simulink library "BWB_library"  (R2017b)
settings: Solver=VariableStepAuto  StartTime=0.0  StopTime=10.0  RelTol=1e-3
undefined symbols (not defined in the file or in its folder): BWB, BWB_uncoupled, BWBlat, BWBlat1, BWBlon, F, I, Ixx, Iyy, Izz, Light, m, MIL, pqr0, ptp0, Vb0, x0, Xe0
libraries: aerolibasang x4, aerolibwind2 x3, shared6dof x2, aerolibadyn x2, aerolibatmos2 x1
(part 1 of 2)
settings Model: Creator=Liam Uni  LastModifiedBy=Liam Uni

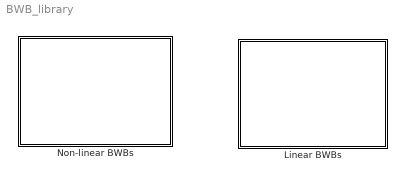
== system BWB_library ==
  Linear BWBs : Subsystem
      mask Display:
      | image('bwb.jpg');
      | 
      | disp('Linear')
  Non-linear BWBs : Subsystem
      mask Display:
      | image('bwb.jpg');
      | 
      | disp('Non-linear')

== system BWB_library/Linear BWBs ==
  BWB lateral : Subsystem  mask{x0=x0}
      mask prompts: x0 "Intial Conditions"
      mask init:
      | open('BWBss')
      mask DialogControl DescGroupVar Prompt: BWB lateral no engine
      mask DialogControl DescTextVar Prompt: Linear model of BWB's lateral dynamics, y(t)=[V p r phi psi] . 12 flaps.
      mask Display:
      | image('bwb.jpg');
      | port_label('input', 1, 'u(t)');
      | port_label('output', 1, 'y(t)');
  BWB lateral no engine : Subsystem  mask{x0=x0}
      mask prompts: x0 "Intial Conditions"
      mask init:
      | open('BWBss')
      mask DialogControl DescGroupVar Prompt: BWB lateral no engine
      mask DialogControl DescTextVar Prompt: Linear model of BWB's lateral dynamics, y(t)=[V p r phi psi] . 12 flaps.
      mask Display:
      | image('bwb.jpg');
      | port_label('input', 1, 'u(t)');
      | port_label('output', 1, 'y(t)');
  BWB linear : Subsystem  mask{x0=x0}
      mask prompts: x0 "Intial Conditions"
      mask init:
      | open('BWBss')
      mask DialogControl DescGroupVar Prompt: BWB linear
      mask DialogControl DescTextVar Prompt: Full State linear BWB, y(t)=[V p r phi psi U w q theta H]. 15 control inputs, 3 engines and 12 flaps
      mask Display:
      | image('bwb.jpg');
      | port_label('input', 1, 'u(t)');
      | port_label('output', 1, 'y(t)');
  BWB longitudinal : Subsystem  mask{x0=x0}
      mask prompts: x0 "Intial Conditions"
      mask init:
      | open('BWBss')
      mask DialogControl DescGroupVar Prompt: BWB longitudinal
      mask DialogControl DescTextVar Prompt: Linear model of BWB's longitudinal dynamics, y(t)=[U w q theta H] . 15 control inputs, 3 engines and 12 flaps.
      mask Display:
      | image('bwb.jpg');
      | port_label('input', 1, 'u(t)');
      | port_label('output', 1, 'y(t)');
  BWB longitudinal 1 engine : Subsystem  mask{x0=x0}
      mask prompts: x0 "Intial Conditions"
      mask init:
      | open('BWBss')
      mask DialogControl DescGroupVar Prompt: BWB longitudinal 1 engine
      mask DialogControl DescTextVar Prompt: Linear model of BWB's longitudinal dynamics, y(t)=[U w q theta H] . 13 control inputs, 1 engine and 12 flaps.
      mask Display:
      | image('bwb.jpg');
      | port_label('input', 1, 'u(t)');
      | port_label('output', 1, 'y(t)');
  BWB uncoupled : Subsystem  mask{x0=x0}
      mask prompts: x0 "Intial Conditions"
      mask init:
      | open('BWBss')
      mask DialogControl DescGroupVar Prompt: BWB linear uncoupled
      mask DialogControl DescTextVar Prompt: Full State linear BWB, y(t)=[V p r phi psi U w q theta H]. 15 control inputs, 3 engines and 12 flaps. Coupling terms between lateral and longitudinal dynamics are negated
      mask Display:
      | image('bwb.jpg');
      | port_label('input', 1, 'u(t)');
      | port_label('output', 1, 'y(t)');

== system BWB_library/Non-linear BWBs ==
  BWB non-linear : Subsystem  mask{Xe0=Xe0, Vb0=Vb0, ptp0=ptp0, pqr0=pqr0, m=m, I=I}
      mask prompts: Xe0 "Initial position in inertial axes [Xe, Ye, Ze]:"; Vb0 "Initial velocity in body axes [U,v,w]:"; ptp0 "Initial Euler orinetation [phi, theta, psi]:"; pqr0 "Initial body rotation rates [p,q,r]:"; m "Initial mass:"; I "Inertial matrix:"
      mask init:
      | % Mean Earth Radius
      | re=6371E3;
      | 
      | % Gravity 
      | g0=9.80665;
      | 
      | a=343;
      | 
      | Rho= 0.85;
      | 
      | %Gross Area/ m^2
      | Sgross= 1390.6;
      | 
      | %Sref/ m^2
      | Sref=   841.7;
      | 
      | %Wing span/ m
      | b=      80;
      | 
      | %Mean aerodynamic chord/ m
      | cbar=   12.31;
      | 
      | %Trapezoidal aspect ratio
      | AR=     7.14;
      | 
      | %Root chord/ m
      | Croot=  48;
      | 
      | %Tip chord/ m
      | Ctip=   4;
      | 
      | %CoG/ m
      | CoG=    29.4;
      | 
      | %Distance of engines from centre/m
      | Deng=5;
      | 
      | %Length of Aircraft/m
      | Length=50.9;
      | 
      | %% Normal Force Coefficient 
      | 
      | Cz0=    0.0217;
      | Czalf=  -5.4868;
      | Czf1=   -0.4866;
      | Czf2=   -0.1602;
      | Czf3=   -0.2222;
      | Czf4=   -0.2274;
      | Czf5=   -0.1042;
      | Czq=    -1.0787;
      | 
      | %% Axial Force Coefficient
      | 
      | Cx0=    0.0117;
      | Cx1=    -0.0200;
      | Cx2=    0.1200;
      | 
      | %% Side Force Coefficient
      | 
      | Cybet0=     -0.3086;
      | Cybetalf=   0.4879;
      | Cyp0=       -0.0814;
      | Cypalf=     2.0666;
      | Cyf1=       -0.0092;
      | Cyf2=       -0.0060;
      | Cyf3=       -0.0088;
      | Cyf4=       -0.0154;
      | Cyf5=       -0.0184;
      | Cydr=       0.0467;
      | Cyr=        -0.1555;
      | 
      | %% Roll Moment Coefficient
      | 
      | Clbet0=     -0.0465;
      | Clbetalf=   -0.3007;
      | Clp0=       -0.3562;
      | Clpalf=     0.0735;
      | Clf1=       -0.0274;
      | Clf2=       -0.0230;
      | Clf3=       -0.0442;
      | Clf4=       -0.0644;
      | Clf5=       -0.0396;
      | Cldr=       0.0156;
      | Clr0=       0.0272;
      | Clralf=     0.5867;
      | 
      | %% Pitch Moment Coefficient
      | 
      | Cm0=        -0.0370;
      | Cmalf=      -0.9950;
      | Cmq=        -0.8799;
      | Cmf1=       -0.3562;
      | Cmf2=       -0.1046;
      | Cmf3=       -0.1432;
      | Cmf4=       -0.1944;
      | Cmf5=       -0.1238;
      | 
      | %% Yaw Moment Coefficient
      | 
      | Cnbet0=    0.0152;
      | Cnbetalf=  -0.2787;
      | Cnp0=       0.0134;
      | Cnpalf=     -0.8733;
      | Cnr0=       -0.0315;
      | Cnralf=     0.0867;
      | Cnf1=       0.0016;
      | Cnf2=       0.0012;
      | Cnf3=       0.0014;
      | Cnf4=       0.0028;
      | Cnf5=       0.0042;
      | Cndr=       -0.0155;
      mask DialogControl DescGroupVar Prompt: BWB non-linear
      mask DialogControl DescTextVar Prompt: Non-linear full state linear BWB, y(t)=[V p r phi psi U w q theta H]. 15 control inputs, 3 engines and 12 flaps. With simplified environment
      mask Display:
      | image('bwb.jpg');
      | port_label('input', 1, 'u(t)');
      | port_label('output', 1, 'y(t)');
  BWB w/ environment : Subsystem  mask{Xe0=Xe0, Vb0=Vb0, ptp0=ptp0, pqr0=pqr0, m=m, I=I}
      mask prompts: Xe0 "Initial position in inertial axes [Xe, Ye, Ze]:"; Vb0 "Initial velocity in body axes [U,v,w]:"; ptp0 "Initial Euler orinetation [phi, theta, psi]:"; pqr0 "Initial body rotation rates [p,q,r]:"; m "Initial mass:"; I "Inertial matrix:"
      mask init:
      | %Gross Area/ m^2
      | Sgross= 1390.6;
      | 
      | %Sref/ m^2
      | Sref=   841.7;
      | 
      | %Wing span/ m
      | b=      80;
      | 
      | %Mean aerodynamic chord/ m
      | cbar=   12.31;
      | 
      | %Trapezoidal aspect ratio
      | AR=     7.14;
      | 
      | %Root chord/ m
      | Croot=  48;
      | 
      | %Tip chord/ m
      | Ctip=   4;
      | 
      | %CoG/ m
      | CoG=    29.4;
      | 
      | %Distance of engines from centre/m
      | Deng=5;
      | 
      | %Length of Aircraft/m
      | Length=50.9;
      | 
      | %% Normal Force Coefficient 
      | 
      | Cz0=    0.0217;
      | Czalf=  -5.4868;
      | Czf1=   -0.4866;
      | Czf2=   -0.1602;
      | Czf3=   -0.2222;
      | Czf4=   -0.2274;
      | Czf5=   -0.1042;
      | Czq=    -1.0787;
      | 
      | %% Axial Force Coefficient
      | 
      | Cx0=    0.0117;
      | Cx1=    -0.0200;
      | Cx2=    0.1200;
      | 
      | %% Side Force Coefficient
      | 
      | Cybet0=     -0.3086;
      | Cybetalf=   0.4879;
      | Cyp0=       -0.0814;
      | Cypalf=     2.0666;
      | Cyf1=       -0.0092;
      | Cyf2=       -0.0060;
      | Cyf3=       -0.0088;
      | Cyf4=       -0.0154;
      | Cyf5=       -0.0184;
      | Cydr=       0.0467;
      | Cyr=        -0.1555;
      | 
      | %% Roll Moment Coefficient
      | 
      | Clbet0=     -0.0465;
      | Clbetalf=   -0.3007;
      | Clp0=       -0.3562;
      | Clpalf=     0.0735;
      | Clf1=       -0.0274;
      | Clf2=       -0.0230;
      | Clf3=       -0.0442;
      | Clf4=       -0.0644;
      | Clf5=       -0.0396;
      | Cldr=       0.0156;
      | Clr0=       0.0272;
      | Clralf=     0.5867;
      | 
      | %% Pitch Moment Coefficient
      | 
      | Cm0=        -0.0370;
      | Cmalf=      -0.9950;
      | Cmq=        -0.8799;
      | Cmf1=       -0.3562;
      | Cmf2=       -0.1046;
      | Cmf3=       -0.1432;
      | Cmf4=       -0.1944;
      | Cmf5=       -0.1238;
      | 
      | %% Yaw Moment Coefficient
      | 
      | Cnbet0=    0.0152;
      | Cnbetalf=  -0.2787;
      | Cnp0=       0.0134;
      | Cnpalf=     -0.8733;
      | Cnr0=       -0.0315;
      | Cnralf=     0.0867;
      | Cnf1=       0.0016;
      | Cnf2=       0.0012;
      | Cnf3=       0.0014;
      | Cnf4=       0.0028;
      | Cnf5=       0.0042;
      | Cndr=       -0.0155;
      mask DialogControl DescGroupVar Prompt: BWB w/ environment
      mask DialogControl DescTextVar Prompt: Non-linear full state linear BWB, y(t)=[V p r phi psi U w q theta H]. 15 control inputs, 3 engines and 12 flaps. With realistic environment
      mask Display:
      | image('bwb.jpg');
      | port_label('input', 1, 'u(t)');
      | port_label('output', 1, 'y(t)');

== system BWB_library/Linear BWBs/BWB lateral ==
  u(t) : Inport
  State-Space : StateSpace  A=BWBlat.A  B=BWBlat.B  C=BWBlat.C  D=BWBlat.D  InitialCondition=x0
  System States : Outport
  wires:
  State-Space/1 -> System States/1
  u(t)/1 -> State-Space/1

== system BWB_library/Linear BWBs/BWB lateral no engine ==
  u(t) : Inport
  State-Space : StateSpace  A=BWBlat1.A  B=BWBlat1.B  C=BWBlat1.C  D=BWBlat1.D  InitialCondition=x0
  System States : Outport
  wires:
  u(t)/1 -> State-Space/1
  State-Space/1 -> System States/1

== system BWB_library/Linear BWBs/BWB linear ==
  u(t) : Inport
  State-Space : StateSpace  A=BWB.A  B=BWB.B  C=BWB.C  D=BWB.D  InitialCondition=x0
  System States : Outport
  wires:
  State-Space/1 -> System States/1
  u(t)/1 -> State-Space/1

== system BWB_library/Linear BWBs/BWB longitudinal ==
  u(t) : Inport
  State-Space : StateSpace  A=BWBlon.A  B=BWBlon.B  C=BWBlon.C  D=BWBlon.D  InitialCondition=x0
  System States : Outport
  wires:
  u(t)/1 -> State-Space/1
  State-Space/1 -> System States/1

== system BWB_library/Linear BWBs/BWB longitudinal 1 engine ==
  u(t) : Inport
  State-Space : StateSpace  A=BWBlon.A  B=BWBlon.B  C=BWBlon.C  D=BWBlon.D  InitialCondition=x0
  System States : Outport
  wires:
  u(t)/1 -> State-Space/1
  State-Space/1 -> System States/1

== system BWB_library/Linear BWBs/BWB uncoupled ==
  u(t) : Inport
  State-Space : StateSpace  A=BWB_uncoupled.A  B=BWB_uncoupled.B  C=BWB_uncoupled.C  D=BWB_uncoupled.D  InitialCondition=x0
  System States : Outport
  wires:
  State-Space/1 -> System States/1
  u(t)/1 -> State-Space/1

== system BWB_library/Non-linear BWBs/BWB non-linear ==
  u(t) : Inport
  6DOF (Euler Angles) : shared6dof/6DOF (Euler Angles)  units=Metric (MKS)  mtype=Fixed  rep=Euler Angles  xme_0=Xe0  Vm_0=Vb0  eul_0=ptp0*0.0174533  pm_0=pqr0*0.0174533  mass_0=m  mass_e=0.5  mass_f=2.0  inertia=diag([Ixx, Iyy, Izz])  inertia_e=eye(3)  inertia_f=2*eye(3)  k_quat=1.0  vre_flag=on  abi_flag=on
      settings: SourceProductBaseCode=AE
  Bus Selector1 : BusSelector  OutputSignals=Vb,phi;theta;psi,pqr,Xe
  Demux : Demux  Outputs=3
  Demux1 : Demux  Outputs=3
  Demux2 : Demux  Outputs=3
  Gain : Gain  Gain=-1
  Model o/p bus : BusCreator  Inputs=6
  Mux : Mux  Inputs=10
  Selector : Selector  InputPortWidth=3  IndexOptions=Index vector (dialog)  Indices=[3]  OutputSizes=1
  Subsystem1 : Subsystem
  Subsystem3 : Subsystem
  Terminator1 : Terminator
  Terminator2 : Terminator
  Terminator3 : Terminator
  System States : Outport
  wires:
  6DOF (Euler Angles)/1 -> Model o/p bus/1  "Ve"
  6DOF (Euler Angles)/7 -> Terminator2/1
  6DOF (Euler Angles)/9 -> Terminator3/1
  6DOF (Euler Angles)/3 -> Model o/p bus/3  "phi;theta;psi"
  6DOF (Euler Angles)/6 -> Model o/p bus/6  "pqr"
  6DOF (Euler Angles)/4 -> Model o/p bus/4  "DCM"
  6DOF (Euler Angles)/8 -> Terminator1/1
  6DOF (Euler Angles)/5 -> Model o/p bus/5  "Vb"
  6DOF (Euler Angles)/2 -> Model o/p bus/2  "Xe"
  Subsystem3/1(Forces) -> 6DOF (Euler Angles)/1
  Subsystem3/2(Moments) -> 6DOF (Euler Angles)/2
  Subsystem1/1(Environment) -> Subsystem3/2(Environment)
  u(t)/1 -> Subsystem3/1(ud(t))
  Bus Selector1/2 -> Demux1/1  "<phi;theta;psi>"
  Mux/1 -> System States/1
  Demux/1 -> Mux/6
  Demux2/2 -> Mux/8
  Demux2/3 -> Mux/3
  Bus Selector1/3 -> Demux2/1  "<pqr>"
  Bus Selector1/1 -> Demux/1  "<Vb>"
  Model o/p bus/1 -> Bus Selector1/1, Subsystem1/1(System States)
  Demux/3 -> Mux/7
  Demux1/3 -> Mux/5
  Gain/1 -> Mux/10
  Demux1/1 -> Mux/4
  Demux2/1 -> Mux/2
  Demux/2 -> Mux/1
  Demux1/2 -> Mux/9
  Selector/1 -> Gain/1
  Bus Selector1/4 -> Selector/1  "<Xe>"

== system BWB_library/Non-linear BWBs/BWB w// environment ==
  u(t) : Inport
  6DOF (Euler Angles) : shared6dof/6DOF (Euler Angles)  units=Metric (MKS)  mtype=Fixed  rep=Euler Angles  xme_0=Xe0  Vm_0=Vb0  eul_0=ptp0*0.0174533  pm_0=pqr0*0.0174533  mass_0=m  mass_e=0.5  mass_f=2.0  inertia=diag([Ixx, Iyy, Izz])  inertia_e=eye(3)  inertia_f=2*eye(3)  k_quat=1.0  vre_flag=on  abi_flag=on
      settings: SourceProductBaseCode=AE
  Bus Selector1 : BusSelector  OutputSignals=Vb,phi;theta;psi,pqr,Xe
  Demux : Demux  Outputs=3
  Demux1 : Demux  Outputs=3
  Demux2 : Demux  Outputs=3
  Gain : Gain  Gain=-1
  Model o/p bus : BusCreator  Inputs=6
  Mux : Mux  Inputs=10
  Selector : Selector  InputPortWidth=3  IndexOptions=Index vector (dialog)  Indices=[3]  OutputSizes=1
  Subsystem1 : Subsystem
  Subsystem3 : Subsystem
  Terminator1 : Terminator
  Terminator2 : Terminator
  Terminator3 : Terminator
  System States : Outport
  wires:
  6DOF (Euler Angles)/1 -> Model o/p bus/1  "Ve"
  6DOF (Euler Angles)/7 -> Terminator2/1
  6DOF (Euler Angles)/9 -> Terminator3/1
  6DOF (Euler Angles)/3 -> Model o/p bus/3  "phi;theta;psi"
  6DOF (Euler Angles)/6 -> Model o/p bus/6  "pqr"
  6DOF (Euler Angles)/4 -> Model o/p bus/4  "DCM"
  6DOF (Euler Angles)/8 -> Terminator1/1
  6DOF (Euler Angles)/5 -> Model o/p bus/5  "Vb"
  6DOF (Euler Angles)/2 -> Model o/p bus/2  "Xe"
  Subsystem3/1(Forces) -> 6DOF (Euler Angles)/1
  Subsystem3/2(Moments) -> 6DOF (Euler Angles)/2
  Subsystem1/1(Environment) -> Subsystem3/2(Environment)
  u(t)/1 -> Subsystem3/1(ud(t))
  Bus Selector1/2 -> Demux1/1  "<phi;theta;psi>"
  Demux2/3 -> Mux/3
  Demux2/1 -> Mux/2
  Model o/p bus/1 -> Bus Selector1/1, Subsystem1/1(System States)
  Demux2/2 -> Mux/8
  Demux1/2 -> Mux/9
  Bus Selector1/1 -> Demux/1  "<Vb>"
  Bus Selector1/3 -> Demux2/1  "<pqr>"
  Demux1/1 -> Mux/4
  Demux/2 -> Mux/1
  Demux/3 -> Mux/7
  Demux/1 -> Mux/6
  Demux1/3 -> Mux/5
  Bus Selector1/4 -> Selector/1  "<Xe>"
  Selector/1 -> Gain/1
  Mux/1 -> System States/1
  Gain/1 -> Mux/10

== system BWB_library/Non-linear BWBs/BWB non-linear/Subsystem1 ==
  System States : Inport
  Abs : Abs
  Bus Creator : BusCreator  Inputs=7
  Bus Selector1 : BusSelector  OutputSignals=Xe,phi;theta;psi,DCM,Vb,pqr
  Constant : Constant  Value=0
  Constant2 : Constant  Value=Rho
  Gain : Gain  Gain=0.5
  Gravity in Earth Axes : Gain  Gain=m  SaturateOnIntegerOverflow=on  OutDataTypeStr=Inherit: Same as input  ParamDataTypeStr=Inherit: Same as input
  Height : Selector  InputPortWidth=3  IndexOptions=Index vector (dialog)  Indices=[3]  OutputSizes=1
  "Incidence, Sideslip, & Airspeed" : aerolibasang/Incidence, Sideslip, & Airspeed
      settings: SourceProductName=Aerospace Blockset
  Inertial to Body : Product  Multiplication=Matrix(*)  SaturateOnIntegerOverflow=on  InputSameDT=on  OutDataTypeStr=Inherit: Same as first input
  Math Function : Math  Operator=square  SaturateOnIntegerOverflow=on
  Mux : Mux  Inputs=3
  Mux1 : Mux  Inputs=2
  Product : Product
  Selector : Selector  InputPortWidth=3  IndexOptions=Index vector (dialog)  Indices=[3]  OutputSizes=1
  Subsystem1 : Subsystem
  z-->h : Abs  SaturateOnIntegerOverflow=on
  Environment : Outport
  wires:
  Bus Selector1/3 -> Inertial to Body/1  "<DCM>"
  Bus Selector1/2 -> Bus Creator/3  "<phi;theta;psi>"
  Bus Creator/1 -> Environment/1
  Selector/1 -> Abs/1
  Abs/1 -> Bus Creator/7  "Altitude"
  z-->h/1 -> Subsystem1/1(Height)
  Gain/1 -> Product/1
  Product/1 -> Bus Creator/6  "qbar"
  Constant/1 -> Mux/1, Mux/2
  Gravity in Earth Axes/1 -> Mux/3
  Math Function/1 -> Product/2
  Constant2/1 -> Gain/1  "rho"
  Bus Selector1/1 -> Height/1, Selector/1  "<Xe>"
  Height/1 -> z-->h/1
  Mux/1 -> Inertial to Body/2
  Subsystem1/1(g) -> Gravity in Earth Axes/1
  Inertial to Body/1 -> Bus Creator/2  "Fg"
  Bus Selector1/4 -> "Incidence, Sideslip, & Airspeed"/1  "<Vb>"
  Bus Selector1/5 -> Bus Creator/1  "<pqr>"
  "Incidence, Sideslip, & Airspeed"/1 -> Mux1/1
  "Incidence, Sideslip, & Airspeed"/2 -> Mux1/2
  Mux1/1 -> Bus Creator/5  "Incid"
  "Incidence, Sideslip, & Airspeed"/3 -> Bus Creator/4, Math Function/1  "V"
  System States/1 -> Bus Selector1/1

== system BWB_library/Non-linear BWBs/BWB non-linear/Subsystem3 ==
  ud(t) : Inport
  Environment : Inport  Port=2
  Bus Selector : BusSelector  OutputSignals=Incid,V,pqr,qbar,Fg
  Forces and Moments : Subsystem  AncestorBlock=aeroblk_lib_HL20/HL20 Airframe/Forces and Moments
  Subsystem : Subsystem
  Subsystem2 : Subsystem
  Sum : Sum  Inputs=|++  SaturateOnIntegerOverflow=on  InputSameDT=on  OutDataTypeStr=Inherit: Same as first input
  Forces : Outport
  Moments : Outport  Port=2
  wires:
  ud(t)/1 -> Subsystem2/1(Control Inputs)
  Bus Selector/5 -> Sum/2  "<Fg>"
  Subsystem/1(Aerodynamic Coeffs) -> Forces and Moments/1(Coeff)
  Forces and Moments/1(X,Y,Z) -> Sum/1
  Forces and Moments/2(LMN) -> Moments/1
  Sum/1 -> Forces/1
  Environment/1 -> Bus Selector/1
  Bus Selector/1 -> Subsystem/2(incid)  "<Incid>"
  Bus Selector/2 -> Subsystem/3(V)  "<V>"
  Bus Selector/3 -> Subsystem/4(pqr)  "<pqr>"
  Bus Selector/4 -> Forces and Moments/3(qbar)  "<qbar>"
  Subsystem2/1(Aerodynamic Controls) -> Subsystem/1(u(t))
  Subsystem2/2(Engine Controls) -> Forces and Moments/2(Thrust)

== system BWB_library/Non-linear BWBs/BWB w// environment/Subsystem1 ==
  System States : Inport
  Abs : Abs
  Alpha,Beta,Mach1 : Subsystem
  Bus Creator : BusCreator  Inputs=7
  Bus Selector1 : BusSelector  OutputSignals=Ve,Xe,phi;theta;psi,DCM,Vb,pqr
  Environment Models1 : Subsystem
  Selector : Selector  InputPortWidth=3  IndexOptions=Index vector (dialog)  Indices=[3]  OutputSizes=1
  Environment : Outport
  wires:
  Alpha,Beta,Mach1/3(V) -> Bus Creator/4  "V"
  Alpha,Beta,Mach1/2("p,q,r ") -> Bus Creator/3  "pqr"
  Bus Selector1/6 -> Alpha,Beta,Mach1/6(p,q,r)  "<pqr>"
  Bus Selector1/2 -> Selector/1, Environment Models1/2(Xe)  "<Xe>"
  Alpha,Beta,Mach1/4(Mach) -> Bus Creator/5  "Mach"
  Bus Selector1/1 -> Environment Models1/1(Ve)  "<Ve>"
  Bus Selector1/4 -> Environment Models1/4(DCM)  "<DCM>"
  Environment Models1/4(Air Density) -> Alpha,Beta,Mach1/3(Air Density)
  System States/1 -> Bus Selector1/1
  Environment Models1/2(Speed of Sound) -> Alpha,Beta,Mach1/1(Speed of Sound)
  Bus Selector1/3 -> Environment Models1/3(Euler)  "<phi;theta;psi>"
  Environment Models1/1(Fg) -> Bus Creator/1  "Fg"
  Alpha,Beta,Mach1/1(qbar) -> Bus Creator/2  "qbar"
  Bus Creator/1 -> Environment/1
  Alpha,Beta,Mach1/5(Incid) -> Bus Creator/6  "Incid"
  Environment Models1/5(Wind Angular Rates) -> Alpha,Beta,Mach1/4(Wind Angular Rates)
  Bus Selector1/5 -> Alpha,Beta,Mach1/5(Vb)  "<Vb>"
  Environment Models1/3(Wind Velocity) -> Alpha,Beta,Mach1/2(Wind Velocity)
  Selector/1 -> Abs/1
  Abs/1 -> Bus Creator/7  "Altitude"

== system BWB_library/Non-linear BWBs/BWB w// environment/Subsystem3 ==
  ud(t) : Inport
  Environment : Inport  Port=2
  Bus Selector : BusSelector  OutputSignals=Incid,V,pqr,qbar,Fg
  Forces and Moments : Subsystem  AncestorBlock=aeroblk_lib_HL20/HL20 Airframe/Forces and Moments
  Subsystem : Subsystem
  Subsystem2 : Subsystem
  Sum : Sum  Inputs=|++  SaturateOnIntegerOverflow=on  InputSameDT=on  OutDataTypeStr=Inherit: Same as first input
  Forces : Outport
  Moments : Outport  Port=2
  wires:
  ud(t)/1 -> Subsystem2/1(Control Inputs)
  Bus Selector/5 -> Sum/2  "<Fg>"
  Subsystem/1(Aerodynamic Coeffs) -> Forces and Moments/1(Coeff)
  Forces and Moments/1(X,Y,Z) -> Sum/1
  Forces and Moments/2(LMN) -> Moments/1
  Sum/1 -> Forces/1
  Environment/1 -> Bus Selector/1
  Bus Selector/1 -> Subsystem/2(incid)  "<Incid>"
  Bus Selector/2 -> Subsystem/3(V)  "<V>"
  Bus Selector/3 -> Subsystem/4(pqr)  "<pqr>"
  Bus Selector/4 -> Forces and Moments/3(qbar)  "<qbar>"
  Subsystem2/1(Aerodynamic Controls) -> Subsystem/1(u(t))
  Subsystem2/2(Engine Controls) -> Forces and Moments/2(Thrust)

== system BWB_library/Non-linear BWBs/BWB non-linear/Subsystem1/Subsystem1 ==
  Height : Inport
  Add : Sum
  Constant1 : Constant  Value=re
  Constant3 : Constant  Value=g0
  Divide : Product  Inputs=*/
  Product1 : Product
  Square : Math  Operator=square  RndMeth=Zero  SaturateOnIntegerOverflow=on
  g : Outport
  wires:
  Add/1 -> Divide/2
  Constant1/1 -> Divide/1, Add/1
  Square/1 -> Product1/1
  Divide/1 -> Square/1
  Product1/1 -> g/1
  Constant3/1 -> Product1/2
  Height/1 -> Add/2

== system BWB_library/Non-linear BWBs/BWB non-linear/Subsystem3/Forces and Moments ==
  Coeff : Inport
  Thrust : Inport  Port=2  Unit=N
  qbar : Inport  Port=3  Unit=Pa
  Aerodynamic Forces and Moments : aerolibadyn/Aerodynamic Forces and Moments   inputAxes=Body  outputForceAxes=Body  outputMomentAxes=Body  S=Sref  b=b  cbar=Croot
      settings: SourceProductName=Aerospace Blockset
  Constant1 : Constant  Value=[(CoG+8), 0, 0]'
  Constant3 : Constant  Value=[CoG 0, 0]'
  Subsystem3 : Subsystem
  Sum : Sum  Inputs=++|  SaturateOnIntegerOverflow=on  InputSameDT=on  OutDataTypeStr=Inherit: Same as first input
  Sum1 : Sum  Inputs=++|  SaturateOnIntegerOverflow=on  InputSameDT=on  OutDataTypeStr=Inherit: Same as first input
  X,Y,Z : Outport  Unit=N  InitialOutput=0
  LMN : Outport  Port=2  Unit=N*m  InitialOutput=0
  wires:
  Constant1/1 -> Aerodynamic Forces and Moments/4
  Constant3/1 -> Aerodynamic Forces and Moments/3
  Aerodynamic Forces and Moments/1 -> Sum/2
  Aerodynamic Forces and Moments/2 -> Sum1/2
  Sum/1 -> X,Y,Z/1
  qbar/1 -> Aerodynamic Forces and Moments/2
  Coeff/1 -> Aerodynamic Forces and Moments/1
  Thrust/1 -> Subsystem3/1(Thrust)
  Subsystem3/1(Engine Forces) -> Sum/1
  Sum1/1 -> LMN/1
  Subsystem3/2(Engine Moments) -> Sum1/1

== system BWB_library/Non-linear BWBs/BWB non-linear/Subsystem3/Subsystem ==
  u(t) : Inport
  incid : Inport  Port=2
  V : Inport  Port=3
  pqr : Inport  Port=4
  Demux : Demux  Outputs=2
  Mux : Mux  Inputs=2
  Subsystem3 : Subsystem
  Subsystem4 : Subsystem
  Aerodynamic Coeffs : Outport
  wires:
  u(t)/1 -> Subsystem4/1(u(t)), Subsystem3/1(u(t))
  Subsystem3/1(Force Coefficients) -> Mux/1
  Mux/1 -> Aerodynamic Coeffs/1
  Subsystem4/1(Moment Coefficients) -> Mux/2
  V/1 -> Subsystem4/2(V), Subsystem3/2(V)
  Demux/1 -> Subsystem4/3(Alpha), Subsystem3/3(Alpha)
  Demux/2 -> Subsystem4/4(Beta), Subsystem3/4(Beta)
  pqr/1 -> Subsystem3/5(pqr), Subsystem4/5(pqr)
  incid/1 -> Demux/1

== system BWB_library/Non-linear BWBs/BWB non-linear/Subsystem3/Subsystem2 ==
  Control Inputs : Inport
  Demux : Demux  Outputs=15
  Mux : Mux  Inputs=12
  Mux1 : Mux  Inputs=3
  Aerodynamic Controls : Outport
  Engine Controls : Outport  Port=2
  wires:
  Control Inputs/1 -> Demux/1
  Mux/1 -> Aerodynamic Controls/1
  Demux/9 -> Mux/9
  Demux/7 -> Mux/7
  Demux/8 -> Mux/8
  Demux/12 -> Mux/12
  Demux/1 -> Mux/1
  Demux/10 -> Mux/10
  Demux/11 -> Mux/11
  Demux/3 -> Mux/3
  Demux/6 -> Mux/6
  Demux/4 -> Mux/4
  Demux/2 -> Mux/2
  Demux/5 -> Mux/5
  Demux/13 -> Mux1/1
  Demux/14 -> Mux1/2
  Demux/15 -> Mux1/3
  Mux1/1 -> Engine Controls/1

== system BWB_library/Non-linear BWBs/BWB w// environment/Subsystem1/Alpha,Beta,Mach1 ==
  Speed of Sound : Inport  Unit=m/s
  Wind Velocity : Inport  Port=2  Unit=m/s  PortDimensions=3
  Air Density : Inport  Port=3  Unit=kg/m^3
  Wind Angular Rates : Inport  Port=4  Unit=rad/s  PortDimensions=3
  Vb : Inport  Port=5  Unit=m/second  PortDimensions=3
  p,q,r : Inport  Port=6  Unit=rad/s  PortDimensions=3
  Dynamic Pressure : aerolibasang/Dynamic Pressure
  "Incidence, Sideslip & Airspeed" : aerolibasang/Incidence, Sideslip, & Airspeed
      settings: SourceProductName=Aerospace Blockset
  Mach Number : aerolibasang/Mach Number
      settings: SourceProductName=Aerospace Blockset  SourceProductBaseCode=AE
  Mux : Mux  Inputs=2
  Sum : Sum  Inputs=|+-  SaturateOnIntegerOverflow=on  InputSameDT=on  OutDataTypeStr=Inherit: Same as first input
  Sum1 : Sum  Inputs=|++  SaturateOnIntegerOverflow=on  InputSameDT=on  OutDataTypeStr=Inherit: Same as first input
  qbar : Outport  Unit=Pa  InitialOutput=0
  "p,q,r " : Outport  Port=2  Unit=rad/s
  V : Outport  Port=3  Unit=m/s
  Mach : Outport  Port=4
  Incid : Outport  Port=5  Unit=rad
  wires:
  "Incidence, Sideslip & Airspeed"/3 -> V/1
  Dynamic Pressure/1 -> qbar/1
  Air Density/1 -> Dynamic Pressure/2
  Mach Number/1 -> Mach/1
  Sum/1 -> Dynamic Pressure/1, Mach Number/1, "Incidence, Sideslip & Airspeed"/1
  Vb/1 -> Sum/1
  Speed of Sound/1 -> Mach Number/2
  Wind Velocity/1 -> Sum/2
  "Incidence, Sideslip & Airspeed"/2 -> Mux/2  "Beta"
  Mux/1 -> Incid/1
  "Incidence, Sideslip & Airspeed"/1 -> Mux/1  "Alpha"
  p,q,r/1 -> Sum1/1
  Wind Angular Rates/1 -> Sum1/2
  Sum1/1 -> "p,q,r "/1

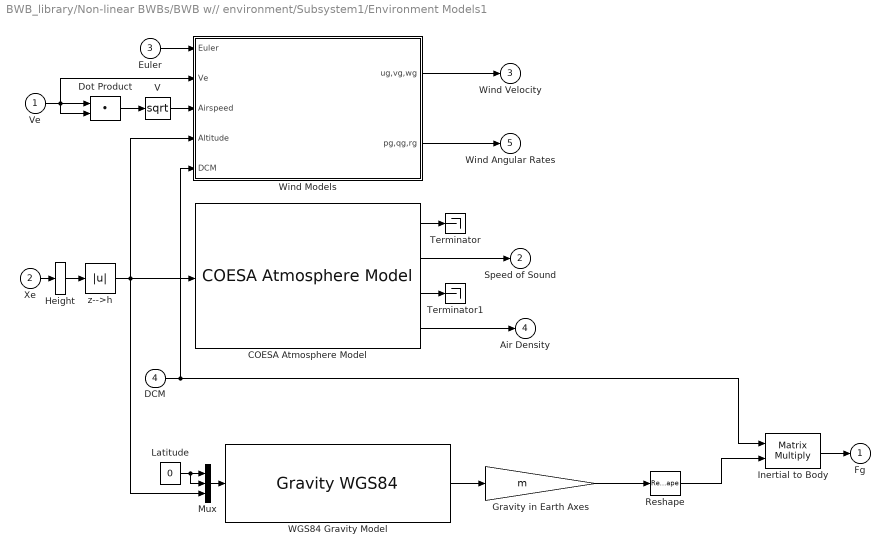
== system BWB_library/Non-linear BWBs/BWB w// environment/Subsystem1/Environment Models1 ==
  Ve : Inport  Unit=m/s
  Xe : Inport  Port=2  Unit=meter  PortDimensions=3
  Euler : Inport  Port=3  Unit=rad
  DCM : Inport  Port=4
  COESA Atmosphere Model : aerolibatmos2/COESA Atmosphere Model  units=Metric (MKS)  spec=1976 COESA-extended U.S. Standard Atmosphere  model=Profile  profile_var=High temperature  profile_percent=10%  profile_alt=5 km (16404 ft)  envelope_var=High temperature  envelope_percent=1%  action=None
  Dot Product : DotProduct  SaturateOnIntegerOverflow=on  OutDataTypeStr=Inherit: Inherit via internal rule
  Gravity in Earth Axes : Gain  Gain=m  SaturateOnIntegerOverflow=on  OutDataTypeStr=Inherit: Same as input  ParamDataTypeStr=Inherit: Same as input
  Height : Selector  InputPortWidth=3  IndexOptions=Index vector (dialog)  Indices=[3]  OutputSizes=1
  Inertial to Body : Product  Multiplication=Matrix(*)  SaturateOnIntegerOverflow=on  InputSameDT=on  OutDataTypeStr=Inherit: Same as first input
  Latitude : Constant  Value=0
  Mux : Mux  Inputs=3
  Reshape : Reshape
  Terminator : Terminator
  Terminator1 : Terminator
  V : Math  Operator=sqrt  SaturateOnIntegerOverflow=on
  "WGS84 Gravity Model  " : GravityWGS84  action=None
  Wind Models : Subsystem
  z-->h : Abs  SaturateOnIntegerOverflow=on
  Fg : Outport  Unit=N  InitialOutput=0
  Speed of Sound : Outport  Port=2  Unit=m/second  InitialOutput=0
  Wind Velocity : Outport  Port=3  Unit=m/second  InitialOutput=0
  Air Density : Outport  Port=4  Unit=kg/m^3  InitialOutput=0
  Wind Angular Rates : Outport  Port=5  Unit=rad/second  InitialOutput=0
  wires:
  Mux/1 -> "WGS84 Gravity Model  "/1
  Euler/1 -> Wind Models/1(Euler)
  Ve/1 -> Dot Product/2, Wind Models/2(Ve), Dot Product/1
  Wind Models/1(ug,vg,wg) -> Wind Velocity/1
  Wind Models/2(pg,qg,rg) -> Wind Angular Rates/1
  Dot Product/1 -> V/1
  z-->h/1 -> Mux/3, COESA Atmosphere Model/1, Wind Models/4(Altitude)
  COESA Atmosphere Model/4 -> Air Density/1
  COESA Atmosphere Model/2 -> Speed of Sound/1
  COESA Atmosphere Model/3 -> Terminator1/1
  COESA Atmosphere Model/1 -> Terminator/1
  Height/1 -> z-->h/1
  Xe/1 -> Height/1
  Latitude/1 -> Mux/2, Mux/1
  "WGS84 Gravity Model  "/1 -> Gravity in Earth Axes/1
  DCM/1 -> Wind Models/5(DCM), Inertial to Body/1
  Inertial to Body/1 -> Fg/1
  V/1 -> Wind Models/3(Airspeed)
  Reshape/1 -> Inertial to Body/2
  Gravity in Earth Axes/1 -> Reshape/1

== system BWB_library/Non-linear BWBs/BWB w// environment/Subsystem3/Forces and Moments ==
  Coeff : Inport
  Thrust : Inport  Port=2  Unit=N
  qbar : Inport  Port=3  Unit=Pa
  Aerodynamic Forces and Moments : aerolibadyn/Aerodynamic Forces and Moments   inputAxes=Body  outputForceAxes=Body  outputMomentAxes=Body  S=Sref  b=b  cbar=Croot
      settings: SourceProductName=Aerospace Blockset
  Constant1 : Constant  Value=[(CoG+8), 0, 0]'
  Constant3 : Constant  Value=[CoG 0, 0]'
  Subsystem3 : Subsystem
  Sum : Sum  Inputs=++|  SaturateOnIntegerOverflow=on  InputSameDT=on  OutDataTypeStr=Inherit: Same as first input
  Sum1 : Sum  Inputs=++|  SaturateOnIntegerOverflow=on  InputSameDT=on  OutDataTypeStr=Inherit: Same as first input
  X,Y,Z : Outport  Unit=N  InitialOutput=0
  LMN : Outport  Port=2  Unit=N*m  InitialOutput=0
  wires:
  Constant1/1 -> Aerodynamic Forces and Moments/4
  Constant3/1 -> Aerodynamic Forces and Moments/3
  Aerodynamic Forces and Moments/1 -> Sum/2
  Aerodynamic Forces and Moments/2 -> Sum1/2
  Sum/1 -> X,Y,Z/1
  qbar/1 -> Aerodynamic Forces and Moments/2
  Coeff/1 -> Aerodynamic Forces and Moments/1
  Thrust/1 -> Subsystem3/1(Thrust)
  Subsystem3/1(Engine Forces) -> Sum/1
  Sum1/1 -> LMN/1
  Subsystem3/2(Engine Moments) -> Sum1/1

== system BWB_library/Non-linear BWBs/BWB w// environment/Subsystem3/Subsystem ==
  u(t) : Inport
  incid : Inport  Port=2
  V : Inport  Port=3
  pqr : Inport  Port=4
  Demux : Demux  Outputs=2
  Mux : Mux  Inputs=2
  Subsystem3 : Subsystem
  Subsystem4 : Subsystem
  Aerodynamic Coeffs : Outport
  wires:
  u(t)/1 -> Subsystem4/1(u(t)), Subsystem3/1(u(t))
  Subsystem3/1(Force Coefficients) -> Mux/1
  Mux/1 -> Aerodynamic Coeffs/1
  Subsystem4/1(Moment Coefficients) -> Mux/2
  V/1 -> Subsystem4/2(V), Subsystem3/2(V)
  Demux/1 -> Subsystem4/3(Alpha), Subsystem3/3(Alpha)
  Demux/2 -> Subsystem4/4(Beta), Subsystem3/4(Beta)
  pqr/1 -> Subsystem3/5(pqr), Subsystem4/5(pqr)
  incid/1 -> Demux/1

== system BWB_library/Non-linear BWBs/BWB w// environment/Subsystem3/Subsystem2 ==
  Control Inputs : Inport
  Demux : Demux  Outputs=15
  Mux : Mux  Inputs=12
  Mux1 : Mux  Inputs=3
  Aerodynamic Controls : Outport
  Engine Controls : Outport  Port=2
  wires:
  Control Inputs/1 -> Demux/1
  Mux/1 -> Aerodynamic Controls/1
  Demux/9 -> Mux/9
  Demux/7 -> Mux/7
  Demux/8 -> Mux/8
  Demux/12 -> Mux/12
  Demux/1 -> Mux/1
  Demux/10 -> Mux/10
  Demux/11 -> Mux/11
  Demux/3 -> Mux/3
  Demux/6 -> Mux/6
  Demux/4 -> Mux/4
  Demux/2 -> Mux/2
  Demux/5 -> Mux/5
  Demux/13 -> Mux1/1
  Demux/14 -> Mux1/2
  Demux/15 -> Mux1/3
  Mux1/1 -> Engine Controls/1

== system BWB_library/Non-linear BWBs/BWB non-linear/Subsystem3/Forces and Moments/Subsystem3 ==
  Thrust : Inport
  Add : Sum  Inputs=+++
  Add1 : Sum
  Constant : Constant  Value=0
  Demux : Demux  Outputs=3
  Gain1 : Gain  Gain=Deng
  Gain2 : Gain  Gain=-Deng
  Mux : Mux  Inputs=3
  Mux1 : Mux  Inputs=3
  Engine Forces : Outport
  Engine Moments : Outport  Port=2
  wires:
  Add/1 -> Mux/1
  Demux/1 -> Add/1, Gain1/1
  Mux/1 -> Engine Forces/1
  Demux/3 -> Gain2/1, Add/3
  Gain2/1 -> Add1/2
  Demux/2 -> Add/2
  Gain1/1 -> Add1/1  "PORT"
  Mux1/1 -> Engine Moments/1
  Thrust/1 -> Demux/1
  Constant/1 -> Mux1/2, Mux1/1, Mux/3, Mux/2
  Add1/1 -> Mux1/3

== system BWB_library/Non-linear BWBs/BWB non-linear/Subsystem3/Subsystem/Subsystem3 ==
  u(t) : Inport
  V : Inport  Port=2
  Alpha : Inport  Port=3
  Beta : Inport  Port=4
  pqr : Inport  Port=5
  Mux : Mux  Inputs=3
  Selector : Selector  InputPortWidth=3  IndexOptions=Index vector (dialog)  Indices=[2]  OutputSizes=1
  Selector1 : Selector  InputPortWidth=3  IndexOptions=Index vector (dialog)  Indices=[3]  OutputSizes=1
  Selector2 : Selector  InputPortWidth=3  IndexOptions=Index vector (dialog)  Indices=[1]  OutputSizes=1
  Subsystem : Subsystem
  Subsystem1 : Subsystem
  Subsystem2 : Subsystem
  Force Coefficients : Outport
  wires:
  Subsystem1/1(Cx) -> Mux/1
  Subsystem2/1(Cy) -> Mux/2
  Mux/1 -> Force Coefficients/1
  Subsystem/1(Cz) -> Mux/3, Subsystem1/1(Cz)
  u(t)/1 -> Subsystem2/6(u(t)), Subsystem/4(u(t))
  V/1 -> Subsystem2/1(True Airspeed), Subsystem/1(True Airspeed)
  Alpha/1 -> Subsystem/2(Angle of Attack), Subsystem2/2(Angle of Attack)
  Beta/1 -> Subsystem2/3(Side Slip Angle)
  pqr/1 -> Selector1/1, Selector2/1, Selector/1
  Selector/1 -> Subsystem/3(Pitch Rate)
  Selector1/1 -> Subsystem2/5(Yaw Rate)
  Selector2/1 -> Subsystem2/4(Roll Rate)

== system BWB_library/Non-linear BWBs/BWB non-linear/Subsystem3/Subsystem/Subsystem4 ==
  u(t) : Inport
  V : Inport  Port=2
  Alpha : Inport  Port=3
  Beta : Inport  Port=4
  pqr : Inport  Port=5
  Mux : Mux  Inputs=3
  Selector : Selector  InputPortWidth=3  IndexOptions=Index vector (dialog)  Indices=[1]  OutputSizes=1
  Selector1 : Selector  InputPortWidth=3  IndexOptions=Index vector (dialog)  Indices=[3]  OutputSizes=1
  Selector2 : Selector  InputPortWidth=3  IndexOptions=Index vector (dialog)  Indices=[2]  OutputSizes=1
  Subsystem : Subsystem
  Subsystem1 : Subsystem
  Subsystem2 : Subsystem
  Moment Coefficients : Outport
  wires:
  Subsystem/1(Cm) -> Mux/2
  Mux/1 -> Moment Coefficients/1
  Subsystem1/1(Cn) -> Mux/3
  Subsystem2/1(Cl) -> Mux/1
  Selector/1 -> Subsystem1/4(Roll Rate), Subsystem2/4(Roll Rate)
  Selector1/1 -> Subsystem2/5(Yaw Rate), Subsystem1/5(Yaw Rate)
  pqr/1 -> Selector1/1, Selector2/1, Selector/1
  V/1 -> Subsystem/1(True Airspeed), Subsystem1/1(True Airspeed), Subsystem2/1(True Airspeed)
  u(t)/1 -> Subsystem2/6(u(t)), Subsystem1/6(u(t)), Subsystem/4(u(t))
  Beta/1 -> Subsystem2/3(Side Slip Angle), Subsystem1/3(Side Slip Angle)
  Alpha/1 -> Subsystem1/2(Angle of Attack), Subsystem/2(Angle of Attack), Subsystem2/2(Angle of Attack)
  Selector2/1 -> Subsystem/3(Pitch Rate)

== system BWB_library/Non-linear BWBs/BWB w// environment/Subsystem1/Environment Models1/Wind Models ==
  Euler : Inport  Unit=rad
  Ve : Inport  Port=2  Unit=m/s
  Airspeed : Inport  Port=3  Unit=m/s
  Altitude : Inport  Port=4  Unit=m
  DCM : Inport  Port=5
  Discrete Wind Gust Model - On : aerolibwind2/Discrete Wind Gust Model  units=Metric (MKS)  Gx=on  Gy=on  Gz=on  t_0=20  d_m=[120 120 80]  v_m=[3.5 3.0 3.0]
      settings: SourceProductName=Aerospace Blockset
  Dryden Wind Turbulence Model (Continuous (+q -r)) : aerolibwind2/Dryden Wind Turbulence Model  (Continuous (+q -r))  units=Metric (MKS)  spec=MIL-F-8785C  model=Continuous Dryden (+q -r)  W20=5  Wdeg=0  TurbProb=10^-2 - Light  L_high=533.4  Wingspan=4  ts=0.1  Seed=[23341 23342 23343 23344]  T_on=on
      settings: SourceProductName=Aerospace Blockset
  Sum : Sum  Inputs=+++  SaturateOnIntegerOverflow=on  InputSameDT=on  OutDataTypeStr=Inherit: Same as first input
  Terminator : Terminator
  Terminator1 : Terminator
  Wind Shear Model : aerolibwind2/Wind Shear Model  units=Metric (MKS)  phase=Category C - Terminal Flight Phase  W_20=1  Wdeg=0
      settings: SourceProductName=Aerospace Blockset
  ug,vg,wg : Outport  Unit=m/s
  pg,qg,rg : Outport  Port=2  Unit=rad/s
  wires:
  Euler/1 -> Terminator1/1
  Ve/1 -> Terminator/1
  Wind Shear Model/1 -> Sum/1
  Dryden Wind Turbulence Model (Continuous (+q -r))/1 -> Sum/2
  Discrete Wind Gust Model - On/1 -> Sum/3
  Sum/1 -> ug,vg,wg/1
  DCM/1 -> Dryden Wind Turbulence Model (Continuous (+q -r))/3, Wind Shear Model/2
  Airspeed/1 -> Dryden Wind Turbulence Model (Continuous (+q -r))/2, Discrete Wind Gust Model - On/1
  Dryden Wind Turbulence Model (Continuous (+q -r))/2 -> pg,qg,rg/1
  Altitude/1 -> Dryden Wind Turbulence Model (Continuous (+q -r))/1, Wind Shear Model/1

== system BWB_library/Non-linear BWBs/BWB w// environment/Subsystem3/Forces and Moments/Subsystem3 ==
  Thrust : Inport
  Add : Sum  Inputs=+++
  Add1 : Sum
  Constant : Constant  Value=0
  Demux : Demux  Outputs=3
  Gain1 : Gain  Gain=Deng
  Gain2 : Gain  Gain=-Deng
  Mux : Mux  Inputs=3
  Mux1 : Mux  Inputs=3
  Engine Forces : Outport
  Engine Moments : Outport  Port=2
  wires:
  Add/1 -> Mux/1
  Demux/1 -> Add/1, Gain1/1
  Mux/1 -> Engine Forces/1
  Demux/3 -> Gain2/1, Add/3
  Gain2/1 -> Add1/2
  Demux/2 -> Add/2
  Gain1/1 -> Add1/1  "PORT"
  Mux1/1 -> Engine Moments/1
  Thrust/1 -> Demux/1
  Constant/1 -> Mux1/2, Mux1/1, Mux/3, Mux/2
  Add1/1 -> Mux1/3

== system BWB_library/Non-linear BWBs/BWB w// environment/Subsystem3/Subsystem/Subsystem3 ==
  u(t) : Inport
  V : Inport  Port=2
  Alpha : Inport  Port=3
  Beta : Inport  Port=4
  pqr : Inport  Port=5
  Mux : Mux  Inputs=3
  Selector : Selector  InputPortWidth=3  IndexOptions=Index vector (dialog)  Indices=[2]  OutputSizes=1
  Selector1 : Selector  InputPortWidth=3  IndexOptions=Index vector (dialog)  Indices=[3]  OutputSizes=1
  Selector2 : Selector  InputPortWidth=3  IndexOptions=Index vector (dialog)  Indices=[1]  OutputSizes=1
  Subsystem : Subsystem
  Subsystem1 : Subsystem
  Subsystem2 : Subsystem
  Force Coefficients : Outport
  wires:
  Subsystem1/1(Cx) -> Mux/1
  Subsystem2/1(Cy) -> Mux/2
  Mux/1 -> Force Coefficients/1
  Subsystem/1(Cz) -> Mux/3, Subsystem1/1(Cz)
  u(t)/1 -> Subsystem2/6(u(t)), Subsystem/4(u(t))
  V/1 -> Subsystem2/1(True Airspeed), Subsystem/1(True Airspeed)
  Alpha/1 -> Subsystem/2(Angle of Attack), Subsystem2/2(Angle of Attack)
  Beta/1 -> Subsystem2/3(Side Slip Angle)
  pqr/1 -> Selector1/1, Selector2/1, Selector/1
  Selector/1 -> Subsystem/3(Pitch Rate)
  Selector1/1 -> Subsystem2/5(Yaw Rate)
  Selector2/1 -> Subsystem2/4(Roll Rate)

== system BWB_library/Non-linear BWBs/BWB w// environment/Subsystem3/Subsystem/Subsystem4 ==
  u(t) : Inport
  V : Inport  Port=2
  Alpha : Inport  Port=3
  Beta : Inport  Port=4
  pqr : Inport  Port=5
  Mux : Mux  Inputs=3
  Selector : Selector  InputPortWidth=3  IndexOptions=Index vector (dialog)  Indices=[1]  OutputSizes=1
  Selector1 : Selector  InputPortWidth=3  IndexOptions=Index vector (dialog)  Indices=[3]  OutputSizes=1
  Selector2 : Selector  InputPortWidth=3  IndexOptions=Index vector (dialog)  Indices=[2]  OutputSizes=1
  Subsystem : Subsystem
  Subsystem1 : Subsystem
  Subsystem2 : Subsystem
  Moment Coefficients : Outport
  wires:
  Subsystem/1(Cm) -> Mux/2
  Mux/1 -> Moment Coefficients/1
  Subsystem1/1(Cn) -> Mux/3
  Subsystem2/1(Cl) -> Mux/1
  Selector/1 -> Subsystem1/4(Roll Rate), Subsystem2/4(Roll Rate)
  Selector1/1 -> Subsystem2/5(Yaw Rate), Subsystem1/5(Yaw Rate)
  pqr/1 -> Selector1/1, Selector2/1, Selector/1
  V/1 -> Subsystem/1(True Airspeed), Subsystem1/1(True Airspeed), Subsystem2/1(True Airspeed)
  u(t)/1 -> Subsystem2/6(u(t)), Subsystem1/6(u(t)), Subsystem/4(u(t))
  Beta/1 -> Subsystem2/3(Side Slip Angle), Subsystem1/3(Side Slip Angle)
  Alpha/1 -> Subsystem1/2(Angle of Attack), Subsystem/2(Angle of Attack), Subsystem2/2(Angle of Attack)
  Selector2/1 -> Subsystem/3(Pitch Rate)

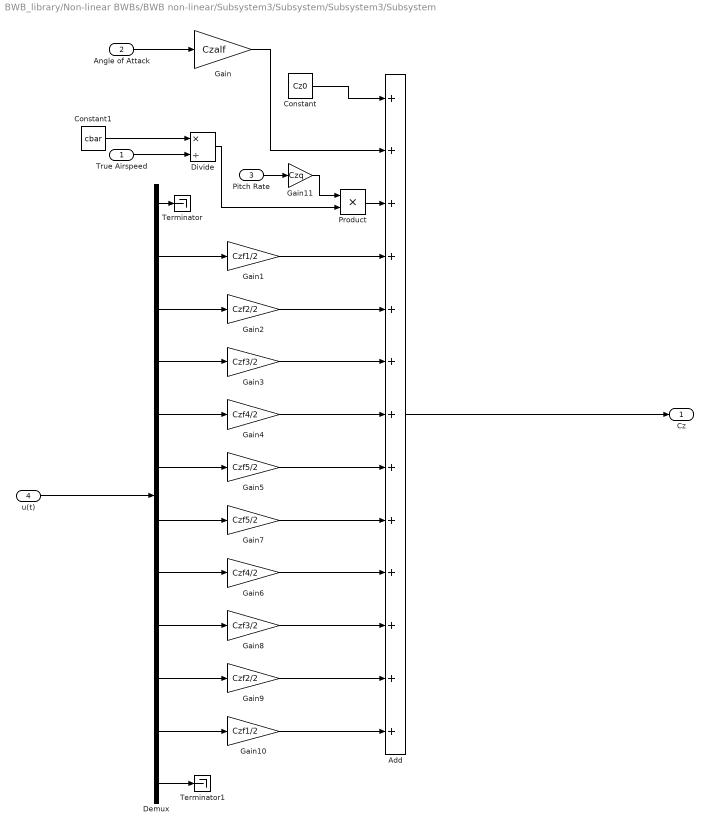
== system BWB_library/Non-linear BWBs/BWB non-linear/Subsystem3/Subsystem/Subsystem3/Subsystem ==
  True Airspeed : Inport
  Angle of Attack : Inport  Port=2
  Pitch Rate : Inport  Port=3
  u(t) : Inport  Port=4
  Add : Sum  Inputs=+++++++++++++
  Constant : Constant  Value=Cz0
  Constant1 : Constant  Value=cbar
  Demux : Demux  Outputs=12
  Divide : Product  Inputs=*/
  Gain : Gain  Gain=Czalf
  Gain1 : Gain  Gain=Czf1/2
  Gain10 : Gain  Gain=Czf1/2
  Gain11 : Gain  Gain=Czq
  Gain2 : Gain  Gain=Czf2/2
  Gain3 : Gain  Gain=Czf3/2
  Gain4 : Gain  Gain=Czf4/2
  Gain5 : Gain  Gain=Czf5/2
  Gain6 : Gain  Gain=Czf4/2
  Gain7 : Gain  Gain=Czf5/2
  Gain8 : Gain  Gain=Czf3/2
  Gain9 : Gain  Gain=Czf2/2
  Product : Product
  Terminator : Terminator
  Terminator1 : Terminator
  Cz : Outport
  wires:
  Add/1 -> Cz/1
  Gain/1 -> Add/2
  True Airspeed/1 -> Divide/2
  Angle of Attack/1 -> Gain/1
  Constant/1 -> Add/1
  Gain9/1 -> Add/12
  Gain7/1 -> Add/9
  Demux/2 -> Gain1/1
  Gain6/1 -> Add/10
  Demux/11 -> Gain10/1
  Demux/6 -> Gain5/1
  Demux/4 -> Gain3/1
  Demux/5 -> Gain4/1
  Divide/1 -> Product/2
  Demux/7 -> Gain7/1
  Gain1/1 -> Add/4
  Gain2/1 -> Add/5
  Gain8/1 -> Add/11
  Gain5/1 -> Add/8
  Demux/8 -> Gain6/1
  Demux/9 -> Gain8/1
  Gain3/1 -> Add/6
  Demux/10 -> Gain9/1
  Demux/3 -> Gain2/1
  Gain10/1 -> Add/13
  Constant1/1 -> Divide/1
  Gain4/1 -> Add/7
  Demux/1 -> Terminator/1
  Demux/12 -> Terminator1/1
  u(t)/1 -> Demux/1
  Gain11/1 -> Product/1
  Pitch Rate/1 -> Gain11/1
  Product/1 -> Add/3

== system BWB_library/Non-linear BWBs/BWB non-linear/Subsystem3/Subsystem/Subsystem3/Subsystem1 ==
  Cz : Inport
  Add : Sum  Inputs=+-+
  Constant : Constant  Value=Cx0
  Gain : Gain  Gain=Cx1
  Gain1 : Gain  Gain=Cx2
  Gain2 : Gain  Gain=-1
  Math Function : Math  Operator=square  SaturateOnIntegerOverflow=on
  Cx : Outport
  wires:
  Math Function/1 -> Gain1/1
  Gain1/1 -> Add/3
  Gain/1 -> Add/2
  Gain2/1 -> Cx/1
  Constant/1 -> Add/1
  Add/1 -> Gain2/1
  Cz/1 -> Math Function/1, Gain/1

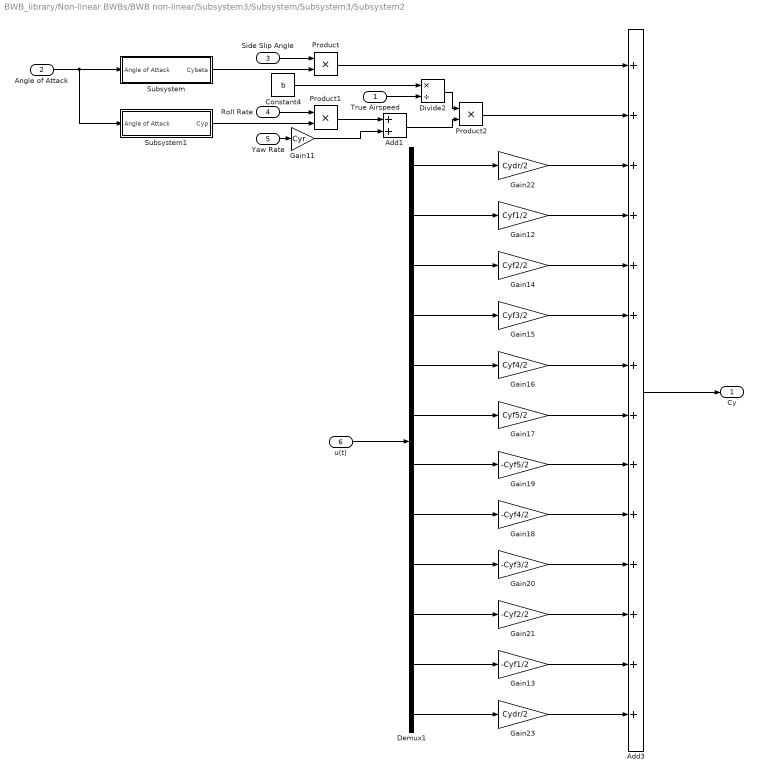
== system BWB_library/Non-linear BWBs/BWB non-linear/Subsystem3/Subsystem/Subsystem3/Subsystem2 ==
  True Airspeed : Inport
  Angle of Attack : Inport  Port=2
  Side Slip Angle : Inport  Port=3
  Roll Rate : Inport  Port=4
  Yaw Rate : Inport  Port=5
  u(t) : Inport  Port=6
  Add1 : Sum
  Add3 : Sum  Inputs=++++++++++++++
  Constant4 : Constant  Value=b
  Demux1 : Demux  Outputs=12
  Divide2 : Product  Inputs=*/
  Gain11 : Gain  Gain=Cyr
  Gain12 : Gain  Gain=Cyf1/2
  Gain13 : Gain  Gain=-Cyf1/2
  Gain14 : Gain  Gain=Cyf2/2
  Gain15 : Gain  Gain=Cyf3/2
  Gain16 : Gain  Gain=Cyf4/2
  Gain17 : Gain  Gain=Cyf5/2
  Gain18 : Gain  Gain=-Cyf4/2
  Gain19 : Gain  Gain=-Cyf5/2
  Gain20 : Gain  Gain=-Cyf3/2
  Gain21 : Gain  Gain=-Cyf2/2
  Gain22 : Gain  Gain=Cydr/2
  Gain23 : Gain  Gain=Cydr/2
  Product : Product
  Product1 : Product
  Product2 : Product
  Subsystem : Subsystem
  Subsystem1 : Subsystem
  Cy : Outport
  wires:
  Side Slip Angle/1 -> Product/1
  Product/1 -> Add3/1
  Angle of Attack/1 -> Subsystem1/1(Angle of Attack), Subsystem/1(Angle of Attack)
  Subsystem/1(Cybeta) -> Product/2
  Subsystem1/1(Cyp) -> Product1/2
  Roll Rate/1 -> Product1/1
  Product1/1 -> Add1/1
  Gain11/1 -> Add1/2
  Yaw Rate/1 -> Gain11/1
  Add1/1 -> Product2/2
  Divide2/1 -> Product2/1
  True Airspeed/1 -> Divide2/2
  Constant4/1 -> Divide2/1
  Product2/1 -> Add3/2
  Demux1/6 -> Gain17/1
  Gain18/1 -> Add3/10
  Demux1/2 -> Gain12/1
  Gain19/1 -> Add3/9
  Demux1/4 -> Gain15/1
  Demux1/7 -> Gain19/1
  Demux1/5 -> Gain16/1
  Demux1/9 -> Gain20/1
  u(t)/1 -> Demux1/1
  Gain15/1 -> Add3/6
  Gain21/1 -> Add3/12
  Demux1/8 -> Gain18/1
  Gain17/1 -> Add3/8
  Gain20/1 -> Add3/11
  Demux1/11 -> Gain13/1
  Gain12/1 -> Add3/4
  Demux1/3 -> Gain14/1
  Demux1/1 -> Gain22/1
  Gain13/1 -> Add3/13
  Gain16/1 -> Add3/7
  Gain14/1 -> Add3/5
  Demux1/10 -> Gain21/1
  Demux1/12 -> Gain23/1
  Gain22/1 -> Add3/3
  Gain23/1 -> Add3/14
  Add3/1 -> Cy/1

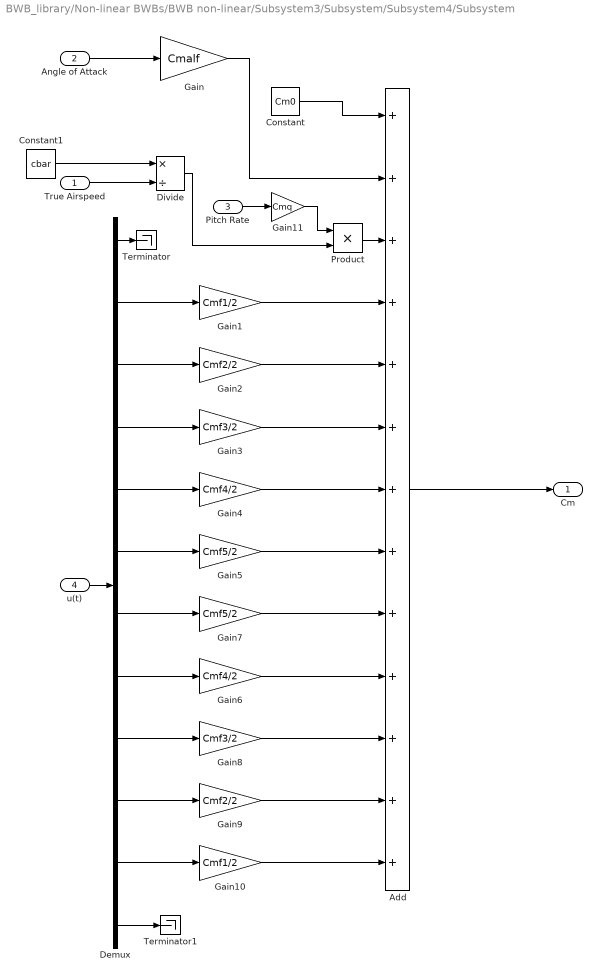
== system BWB_library/Non-linear BWBs/BWB non-linear/Subsystem3/Subsystem/Subsystem4/Subsystem ==
  True Airspeed : Inport
  Angle of Attack : Inport  Port=2
  Pitch Rate : Inport  Port=3
  u(t) : Inport  Port=4
  Add : Sum  Inputs=+++++++++++++
  Constant : Constant  Value=Cm0
  Constant1 : Constant  Value=cbar
  Demux : Demux  Outputs=12
  Divide : Product  Inputs=*/
  Gain : Gain  Gain=Cmalf
  Gain1 : Gain  Gain=Cmf1/2
  Gain10 : Gain  Gain=Cmf1/2
  Gain11 : Gain  Gain=Cmq
  Gain2 : Gain  Gain=Cmf2/2
  Gain3 : Gain  Gain=Cmf3/2
  Gain4 : Gain  Gain=Cmf4/2
  Gain5 : Gain  Gain=Cmf5/2
  Gain6 : Gain  Gain=Cmf4/2
  Gain7 : Gain  Gain=Cmf5/2
  Gain8 : Gain  Gain=Cmf3/2
  Gain9 : Gain  Gain=Cmf2/2
  Product : Product
  Terminator : Terminator
  Terminator1 : Terminator
  Cm : Outport
  wires:
  Add/1 -> Cm/1
  Gain/1 -> Add/2
  True Airspeed/1 -> Divide/2
  Angle of Attack/1 -> Gain/1
  Constant/1 -> Add/1
  Gain9/1 -> Add/12
  Gain7/1 -> Add/9
  Demux/2 -> Gain1/1
  Gain6/1 -> Add/10
  Demux/11 -> Gain10/1
  Demux/6 -> Gain5/1
  Demux/4 -> Gain3/1
  Demux/5 -> Gain4/1
  Divide/1 -> Product/2
  Demux/7 -> Gain7/1
  Gain1/1 -> Add/4
  Gain2/1 -> Add/5
  Gain8/1 -> Add/11
  Gain5/1 -> Add/8
  Demux/8 -> Gain6/1
  Demux/9 -> Gain8/1
  Gain3/1 -> Add/6
  Demux/10 -> Gain9/1
  Demux/3 -> Gain2/1
  Gain10/1 -> Add/13
  Constant1/1 -> Divide/1
  Gain4/1 -> Add/7
  Demux/1 -> Terminator/1
  Demux/12 -> Terminator1/1
  u(t)/1 -> Demux/1
  Gain11/1 -> Product/1
  Pitch Rate/1 -> Gain11/1
  Product/1 -> Add/3

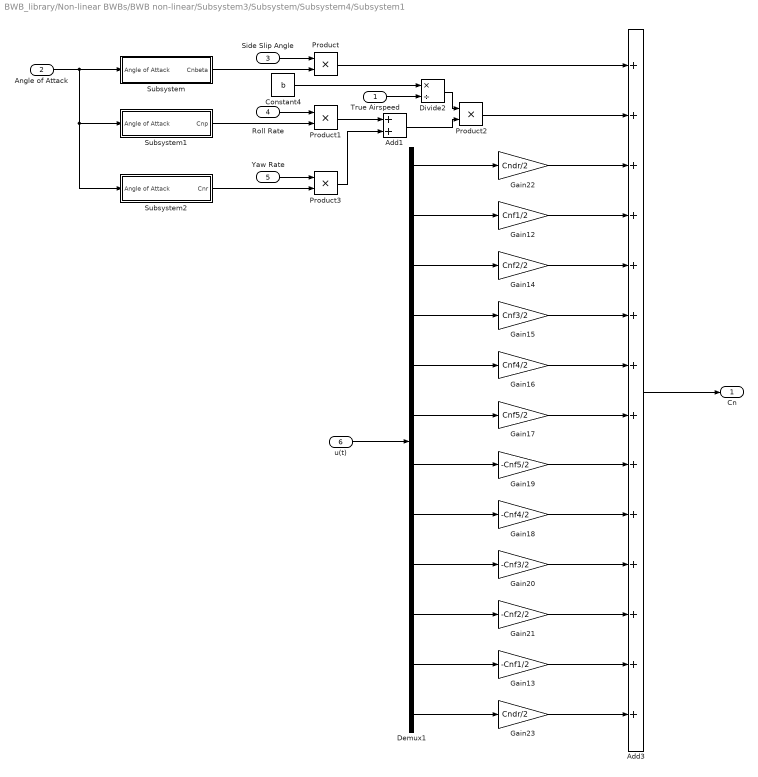
== system BWB_library/Non-linear BWBs/BWB non-linear/Subsystem3/Subsystem/Subsystem4/Subsystem1 ==
  True Airspeed : Inport
  Angle of Attack : Inport  Port=2
  Side Slip Angle : Inport  Port=3
  Roll Rate : Inport  Port=4
  Yaw Rate : Inport  Port=5
  u(t) : Inport  Port=6
  Add1 : Sum
  Add3 : Sum  Inputs=++++++++++++++
  Constant4 : Constant  Value=b
  Demux1 : Demux  Outputs=12
  Divide2 : Product  Inputs=*/
  Gain12 : Gain  Gain=Cnf1/2
  Gain13 : Gain  Gain=-Cnf1/2
  Gain14 : Gain  Gain=Cnf2/2
  Gain15 : Gain  Gain=Cnf3/2
  Gain16 : Gain  Gain=Cnf4/2
  Gain17 : Gain  Gain=Cnf5/2
  Gain18 : Gain  Gain=-Cnf4/2
  Gain19 : Gain  Gain=-Cnf5/2
  Gain20 : Gain  Gain=-Cnf3/2
  Gain21 : Gain  Gain=-Cnf2/2
  Gain22 : Gain  Gain=Cndr/2
  Gain23 : Gain  Gain=Cndr/2
  Product{,1..3} (4 alike) : Product
  Subsystem : Subsystem
  Subsystem1 : Subsystem
  Subsystem2 : Subsystem
  Cn : Outport
  wires:
  Side Slip Angle/1 -> Product/1
  Product/1 -> Add3/1
  Angle of Attack/1 -> Subsystem1/1(Angle of Attack), Subsystem2/1(Angle of Attack), Subsystem/1(Angle of Attack)
  Subsystem/1(Cnbeta) -> Product/2
  Subsystem1/1(Cnp) -> Product1/2
  Roll Rate/1 -> Product1/1
  Product1/1 -> Add1/1
  Product3/1 -> Add1/2
  Yaw Rate/1 -> Product3/1
  Add1/1 -> Product2/2
  Divide2/1 -> Product2/1
  True Airspeed/1 -> Divide2/2
  Constant4/1 -> Divide2/1
  Product2/1 -> Add3/2
  Demux1/6 -> Gain17/1
  Gain18/1 -> Add3/10
  Demux1/2 -> Gain12/1
  Gain19/1 -> Add3/9
  Demux1/4 -> Gain15/1
  Demux1/7 -> Gain19/1
  Demux1/5 -> Gain16/1
  Demux1/9 -> Gain20/1
  u(t)/1 -> Demux1/1
  Gain15/1 -> Add3/6
  Gain21/1 -> Add3/12
  Demux1/8 -> Gain18/1
  Gain17/1 -> Add3/8
  Gain20/1 -> Add3/11
  Demux1/11 -> Gain13/1
  Gain12/1 -> Add3/4
  Demux1/3 -> Gain14/1
  Demux1/1 -> Gain22/1
  Gain13/1 -> Add3/13
  Gain16/1 -> Add3/7
  Gain14/1 -> Add3/5
  Demux1/10 -> Gain21/1
  Demux1/12 -> Gain23/1
  Gain22/1 -> Add3/3
  Gain23/1 -> Add3/14
  Add3/1 -> Cn/1
  Subsystem2/1(Cnr) -> Product3/2

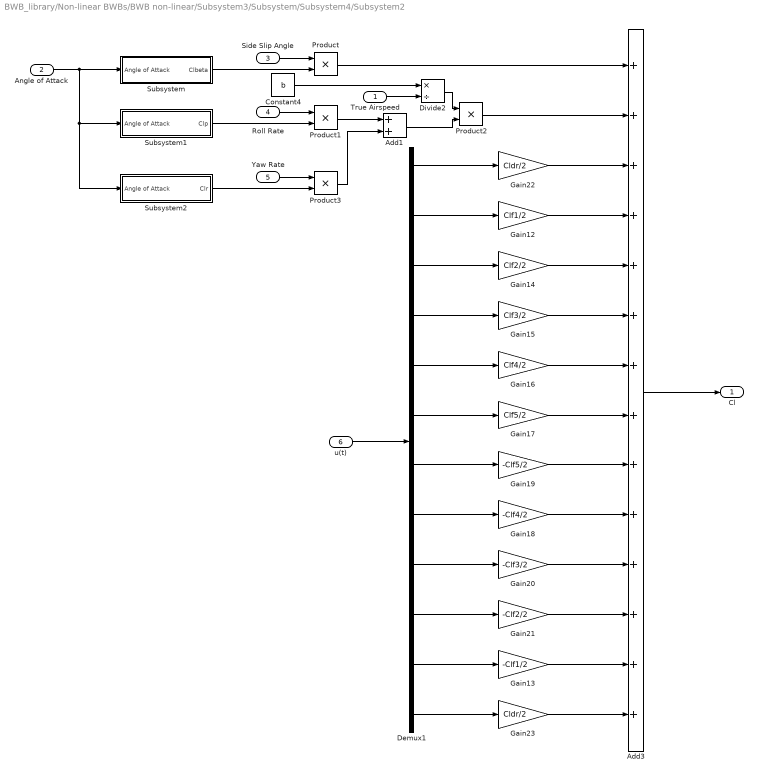
== system BWB_library/Non-linear BWBs/BWB non-linear/Subsystem3/Subsystem/Subsystem4/Subsystem2 ==
  True Airspeed : Inport
  Angle of Attack : Inport  Port=2
  Side Slip Angle : Inport  Port=3
  Roll Rate : Inport  Port=4
  Yaw Rate : Inport  Port=5
  u(t) : Inport  Port=6
  Add1 : Sum
  Add3 : Sum  Inputs=++++++++++++++
  Constant4 : Constant  Value=b
  Demux1 : Demux  Outputs=12
  Divide2 : Product  Inputs=*/
  Gain12 : Gain  Gain=Clf1/2
  Gain13 : Gain  Gain=-Clf1/2
  Gain14 : Gain  Gain=Clf2/2
  Gain15 : Gain  Gain=Clf3/2
  Gain16 : Gain  Gain=Clf4/2
  Gain17 : Gain  Gain=Clf5/2
  Gain18 : Gain  Gain=-Clf4/2
  Gain19 : Gain  Gain=-Clf5/2
  Gain20 : Gain  Gain=-Clf3/2
  Gain21 : Gain  Gain=-Clf2/2
  Gain22 : Gain  Gain=Cldr/2
  Gain23 : Gain  Gain=Cldr/2
  Product{,1..3} (4 alike) : Product
  Subsystem : Subsystem
  Subsystem1 : Subsystem
  Subsystem2 : Subsystem
  Cl : Outport
  wires:
  Side Slip Angle/1 -> Product/1
  Product/1 -> Add3/1
  Angle of Attack/1 -> Subsystem1/1(Angle of Attack), Subsystem2/1(Angle of Attack), Subsystem/1(Angle of Attack)
  Subsystem/1(Clbeta) -> Product/2
  Subsystem1/1(Clp) -> Product1/2
  Roll Rate/1 -> Product1/1
  Product1/1 -> Add1/1
  Product3/1 -> Add1/2
  Yaw Rate/1 -> Product3/1
  Add1/1 -> Product2/2
  Divide2/1 -> Product2/1
  True Airspeed/1 -> Divide2/2
  Constant4/1 -> Divide2/1
  Product2/1 -> Add3/2
  Demux1/6 -> Gain17/1
  Gain18/1 -> Add3/10
  Demux1/2 -> Gain12/1
  Gain19/1 -> Add3/9
  Demux1/4 -> Gain15/1
  Demux1/7 -> Gain19/1
  Demux1/5 -> Gain16/1
  Demux1/9 -> Gain20/1
  u(t)/1 -> Demux1/1
  Gain15/1 -> Add3/6
  Gain21/1 -> Add3/12
  Demux1/8 -> Gain18/1
  Gain17/1 -> Add3/8
  Gain20/1 -> Add3/11
  Demux1/11 -> Gain13/1
  Gain12/1 -> Add3/4
  Demux1/3 -> Gain14/1
  Demux1/1 -> Gain22/1
  Gain13/1 -> Add3/13
  Gain16/1 -> Add3/7
  Gain14/1 -> Add3/5
  Demux1/10 -> Gain21/1
  Demux1/12 -> Gain23/1
  Gain22/1 -> Add3/3
  Gain23/1 -> Add3/14
  Add3/1 -> Cl/1
  Subsystem2/1(Clr) -> Product3/2
